simulink model "Compressor_Heater_Stateflow"  (R2017a)
settings: Solver=VariableStepAuto  StartTime=0.0  StopTime=10.0  RelTol=1e-3
libraries: simulink x2
settings Model: Creator=ACER  LastModifiedBy=peram
settings DataIOCC: ReturnWorkspaceOutputs=on
settings DebuggingCC: UnconnectedInputMsg=none  UnconnectedOutputMsg=none  UnconnectedLineMsg=none  SFMachineParentedDataDiag=error
settings ModelReferenceCC: EnableRefExpFcnMdlSchedulingChecks=off
settings SFSimCC: SimUseLocalCustomCode=on
settings RTWCC: RTWUseLocalCustomCode=on

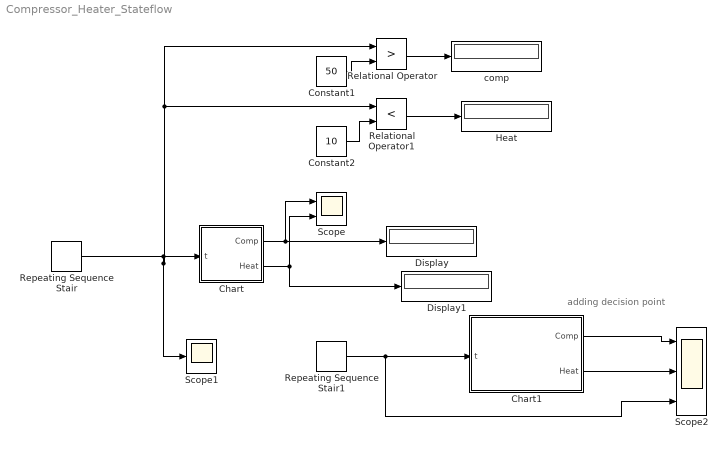
== system Compressor_Heater_Stateflow ==
  note: adding decision point
  Chart : Stateflow chart  TreatAsAtomicUnit=on
  Chart1 : Stateflow chart  TreatAsAtomicUnit=on
  Constant1 : Constant  Value=50
  Constant2 : Constant  Value=10
  Display : Display
  Display1 : Display
  Heat : Display
  Relational Operator : RelationalOperator  Operator=>  OutDataTypeStr=boolean  RndMeth=Simplest
  Relational Operator1 : RelationalOperator  Operator=<  OutDataTypeStr=boolean  RndMeth=Simplest
  Repeating Sequence Stair : simulink/Sources/Repeating Sequence Stair  OutValues=[30 45 50 7 51 0 10 40 60 45 15].'  tsamp=-1  OutMin=[]  OutMax=[]  OutDataTypeStr=double  OutputDataTypeScalingMode=double  OutDataType=fixdt(0,8)  ConRadixGroup=Best Precision: Vector-wise  OutScaling=2^-12
  Repeating Sequence Stair1 : simulink/Sources/Repeating Sequence Stair  OutValues=[ 15 7 55 1].'  tsamp=-1  OutMin=[]  OutMax=[]  OutDataTypeStr=double  OutputDataTypeScalingMode=double  OutDataType=fixdt(0,8)  ConRadixGroup=Best Precision: Vector-wise  OutScaling=2^-12
  Scope : Scope  NumInputPorts=2
  Scope1 : Scope
  Scope2 : Scope  NumInputPorts=3
  comp : Display
  wires:
  Chart/1(Comp) -> Scope/1, Display/1
  Chart/2(Heat) -> Scope/2, Display1/1
  Repeating Sequence Stair/1 -> Relational Operator1/1, Relational Operator/1, Scope1/1, Chart/1(t)
  Constant1/1 -> Relational Operator/2
  Relational Operator/1 -> comp/1
  Relational Operator1/1 -> Heat/1
  Constant2/1 -> Relational Operator1/2
  Chart1/2(Heat) -> Scope2/2
  Repeating Sequence Stair1/1 -> Scope2/3, Chart1/1(t)
  Chart1/1(Comp) -> Scope2/1

== stateflow chart Compressor_Heater_Stateflow/Chart1 ==
  state Default_state
    entry:
    Comp=0;
    Heat = 0;
  state Heater_on
    entry:
    Heat=1;
    during:
    Heat=1;
    exit:
    Heat = 0;
  state Compressor_on
    entry:
    Comp=1;
    during:
    Comp =1;
    exit:
    Comp =0;
  (default) -> (junction 26)
  (junction 26) -> Heater_on [order 1] : [t<10]
  (junction 26) -> Compressor_on [order 2] : [t>50]
  (junction 26) -> Default_state [order 3]
  Default_state -> Heater_on [order 1] : [t<10]
  Heater_on -> Default_state [order 2] : [t>=10||t<50]
  Compressor_on -> Default_state [order 2] : [t>=10||t<50]
  Default_state -> Compressor_on [order 2] : [t>50]
  Heater_on -> Compressor_on [order 1] : [t>50]
  Compressor_on -> Heater_on [order 1] : [t<10]
  data: Comp output; Heat output; t input

== stateflow chart Compressor_Heater_Stateflow/Chart ==
  state Default_state
    entry:
    Comp=0;
    Heat = 0;
  state Heater_on
    entry:
    Heat=1;
    during:
    Heat=1;
    exit:
    Heat = 0;
  state Compressor_on
    entry:
    Comp=1;
    during:
    Comp =1;
    exit:
    Comp =0;
  (default) -> Default_state
  Default_state -> Heater_on [order 1] : [t<10]
  Heater_on -> Default_state [order 2] : [t>=10||t<50]
  Compressor_on -> Default_state [order 2] : [t>=10||t<50]
  Default_state -> Compressor_on [order 2] : [t>50]
  Compressor_on -> Heater_on [order 1] : [t<10]
  Heater_on -> Compressor_on [order 1] : [t>50]
  data: Comp output; Heat output; t input
